simulink model "MBD_week2_prob1"  (R2020b)
settings: Solver=VariableStepAuto  StartTime=0.0  StopTime=10.0  RelTol=1e-3
libraries: simulink_extras x1
settings Model: Creator=varunraj  LastModifiedBy=varunraj

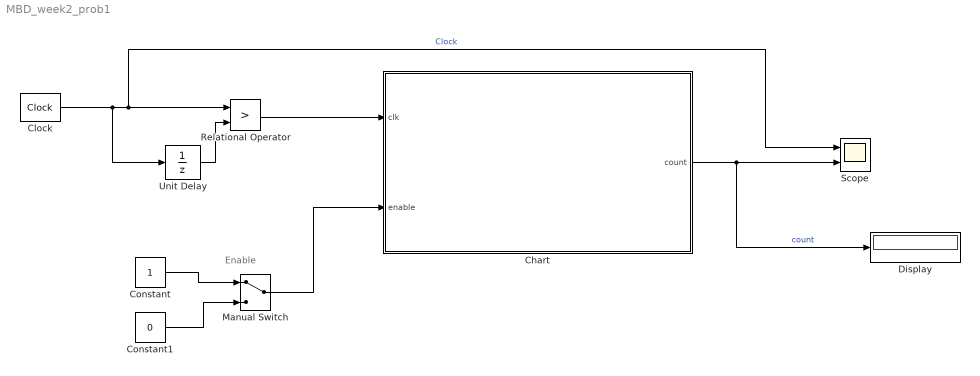
== system MBD_week2_prob1 ==
  note: Enable
  Chart : Stateflow chart  TreatAsAtomicUnit=on
  Clock : simulink_extras/Flip Flops/Clock  period=1
  Constant : Constant
  Constant1 : Constant  Value=0
  Display : Display
  Manual Switch : ManualSwitch
  Relational Operator : RelationalOperator  Operator=>  OutDataTypeStr=boolean  RndMeth=Simplest
  Scope : Scope  NumInputPorts=2
  Unit Delay : UnitDelay  SampleTime=-1  HasFrameUpgradeWarning=on
  wires:
  Relational Operator/1 -> Chart/1(clk)
  Manual Switch/1 -> Chart/2(enable)
  Unit Delay/1 -> Relational Operator/2
  Constant/1 -> Manual Switch/1
  Chart/1(count) -> Display/1, Scope/2  "count"
  Clock/1 -> Scope/1, Relational Operator/1, Unit Delay/1  "Clock"
  Constant1/1 -> Manual Switch/2

== stateflow chart MBD_week2_prob1/Chart ==
  state clock
    en:
    count=0;
  state Counter
    state State1
      en:
      Q3=0;
      Q2=0;
      Q1=0;
    state state5
      en:
      Q3=1;
      Q2=0;
      Q1=0;
    state state2
      en:
      Q3=0;
      Q2=0;
      Q1=1;
    state state4
      en:
      Q3=0;
      Q2=1;
      Q1=1;
    state state3
      en:
      Q3=0;
      Q2=1;
      Q1=0;
    (default) -> State1
    state5 -> State1 : [clk==1]{count=Q3*4+Q2*2+Q1}
    State1 -> state2 : [clk==1]{count=Q3*4+Q2*2+Q1}
    state2 -> state3 : [clk==1]{count=Q3*4+Q2*2+Q1}
    state4 -> state5 : [clk==1]{count=Q3*4+Q2*2+Q1}
    state3 -> state4 : [clk==1]{count=Q3*4+Q2*2+Q1}
  (default) -> clock
  clock -> Counter : [enable==1]{Q3=0;Q2=0;Q1=0;}
  Counter -> clock : [enable==0]{Q3=0;Q2=0;Q1=0}
  data: clk input; count output; enable input; Q3 local; Q2 local; Q1 local
